simulink model "lab2_EmulationPID_Feedforward"  (R2020b)
settings: Solver=VariableStepAuto  StartTime=0.0  StopTime=10.0  RelTol=1e-3
undefined symbols (not defined in the file): BEMF_Compensator, Beq_hat_final, DiscIntNeverNeededParam, drv, enable_BlackBox, friction_Compensator, gbox, inertia_Compensator, Kd, Ki, Kp, mld, mot, rads2rpm, rpm2rads, sens, tau_sf_hat_final, Tl, Ts
libraries: simulink x1
settings Model: Creator=Musta  LastModifiedBy=Musta

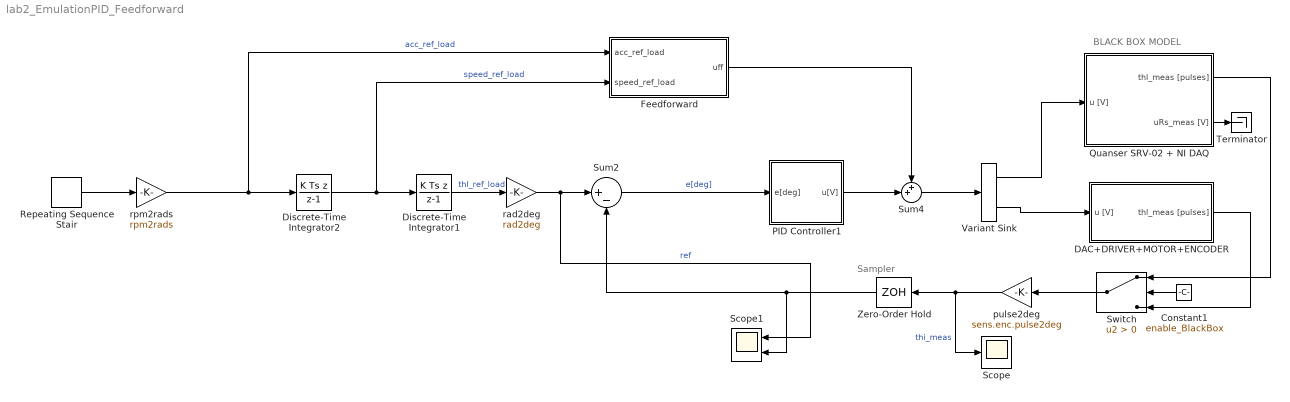
== system lab2_EmulationPID_Feedforward ==
  note: Sampler
  note: BLACK BOX MODEL
  Constant1 : Constant  Value=enable_BlackBox
  DAC+DRIVER+MOTOR+ENCODER : Subsystem
  Discrete-Time Integrator1 : DiscreteIntegrator  IntegratorMethod=Integration: Backward Euler  SampleTime=Ts  ICPrevOutput=DiscIntNeverNeededParam  ICPrevScaledInput=DiscIntNeverNeededParam
  Discrete-Time Integrator2 : DiscreteIntegrator  IntegratorMethod=Integration: Backward Euler  SampleTime=Ts  ICPrevOutput=DiscIntNeverNeededParam  ICPrevScaledInput=DiscIntNeverNeededParam
  Feedforward : Subsystem
  PID Controller1 : Subsystem
  Quanser SRV-02 + NI DAQ : Subsystem  mask(Quanser SRV-02 (with inertial load) + NI DAQ){Ts=Ts, fricType=Karnopp}
      mask prompts: Ts "NI DAQ Sample Time:"; fricType "Friction model"
      mask help: Quanser SRV-02 (with inertial load) + NI DAQ model.
      mask init:
      | %%  Sensors data
      | 
      | %   shunt resistor
      | sens.curr.Rs = 0.5;                         %   resistance [Ohm]   
      | sens.curr.uRs_std = 0.01;                   %   voltage noise standard dev [V]                           
      | sens.curr.uRs_var = sens.curr.uRs_std^2;	%   voltage noise variance [V^2]
      | 
      | %   Hewlett-Packard HEDS-5540#A06 optical encoder
      | sens.enc.ppr = 500*4;                       %   pulses per rotation
      | sens.enc.pulse2deg = 360/sens.enc.ppr;      %   [pulses] -> [deg]
      | sens.enc.pulse2rad = 2*pi/sens.enc.ppr;     %   [pulses] -> [rad]
      | sens.enc.deg2pulse = sens.enc.ppr/360;      %   [deg] -> [pulses]
      | sens.enc.rad2pulse = sens.enc.ppr/2/pi;     %   [rad] -> [pulses]
      | 
      | 
      | %%  Data acquisition board (daq) data
      | 
      | %   NI PCI-6221 DAC data
      | daq.dac.bits = 16;                                  %   resolution (bits)
      | daq.dac.fs   = 10;                                  %   full scale 
      | daq.dac.q    = 2*daq.dac.fs/(2^daq.dac.bits-1);     %	quantization
      | 
      | %   NI PCI-6221 ADC data
      | daq.adc.bits = 16;                                  %   resolution (bits)
      | daq.adc.fs   = 10;                                  %   full scale (as set in SLDRT Analog Input block)
      | daq.adc.q    = 2*daq.adc.fs/(2^daq.adc.bits-1);     %   quantization
      mask Help:
      | Riccardo Antonello (antonello@dei.unipd.it)
      | 
      | April 24, 2020
      | 
      | Dept. of Information Engineering, University of Padova
      mask TypeOptions fricType: Coulomb + viscous | Karnopp
  Repeating Sequence Stair : simulink/Sources/Repeating Sequence Stair  OutValues=[900 0 -900 -900 0 900]  tsamp=0.5  OutMin=[]  OutMax=[]  OutDataTypeStr=double  OutputDataTypeScalingMode=double  OutDataType=fixdt(0,8)  ConRadixGroup=Best Precision: Vector-wise  OutScaling=2^-12
  Scope : Scope
  Scope1 : Scope  NumInputPorts=2
  Sum2 : Sum  Inputs=|+-
  Sum4 : Sum  Inputs=++|
  Switch : Switch  Criteria=u2 > Threshold
  Terminator : Terminator
  Variant Sink : VariantSink
  Zero-Order Hold : ZeroOrderHold  SampleTime=Ts
  pulse2deg : Gain  Gain=sens.enc.pulse2deg
  rad2deg : Gain  Gain=rad2deg
  rpm2rads : Gain  Gain=rpm2rads
  wires:
  PID Controller1/1(u[V]) -> Sum4/2
  Sum2/1 -> PID Controller1/1(e[deg])  "e[deg]"
  Zero-Order Hold/1 -> Scope1/2, Sum2/2
  Feedforward/1(uff) -> Sum4/1
  Discrete-Time Integrator1/1 -> rad2deg/1  "thl_ref_load"
  rpm2rads/1 -> Discrete-Time Integrator2/1, Feedforward/1(acc_ref_load)  "acc_ref_load"
  Discrete-Time Integrator2/1 -> Discrete-Time Integrator1/1, Feedforward/2(speed_ref_load)  "speed_ref_load"
  rad2deg/1 -> Scope1/1, Sum2/1  "ref"
  Repeating Sequence Stair/1 -> rpm2rads/1
  Sum4/1 -> Variant Sink/1
  DAC+DRIVER+MOTOR+ENCODER/1(thl_meas [pulses]) -> Switch/3
  Variant Sink/2 -> DAC+DRIVER+MOTOR+ENCODER/1(u [V])
  Switch/1 -> pulse2deg/1
  Quanser SRV-02 + NI DAQ/1(thl_meas [pulses]) -> Switch/1
  pulse2deg/1 -> Scope/1, Zero-Order Hold/1  "thi_meas"
  Quanser SRV-02 + NI DAQ/2(uRs_meas [V]) -> Terminator/1
  Variant Sink/1 -> Quanser SRV-02 + NI DAQ/1(u [V])
  Constant1/1 -> Switch/2

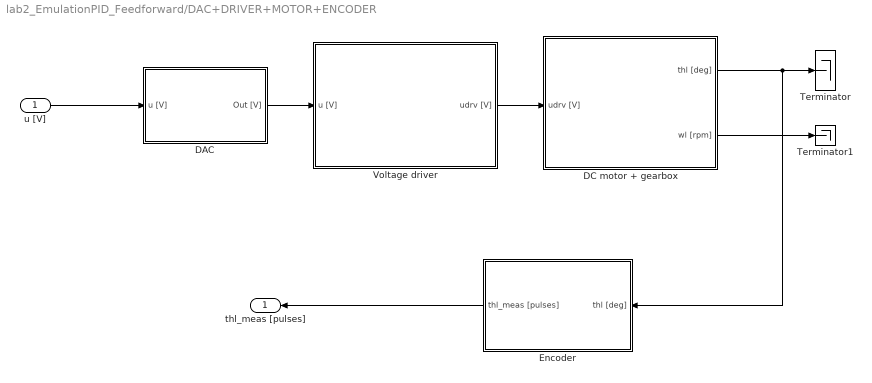
== system lab2_EmulationPID_Feedforward/DAC+DRIVER+MOTOR+ENCODER ==
  u [V] : Inport
  DAC : Subsystem
  DC motor + gearbox : Subsystem
  Encoder : Subsystem
  Terminator : Terminator
  Terminator1 : Terminator
  Voltage driver : Subsystem
  thl_meas [pulses] : Outport
  wires:
  DAC/1(Out [V]) -> Voltage driver/1(u [V])
  DC motor + gearbox/1("thl [deg] ") -> Terminator/1, Encoder/1("thl [deg] ")
  Voltage driver/1(udrv [V]) -> DC motor + gearbox/1(udrv [V])
  DC motor + gearbox/2(wl [rpm]) -> Terminator1/1
  Encoder/1(thl_meas [pulses]) -> thl_meas [pulses]/1
  u [V]/1 -> DAC/1(u [V])

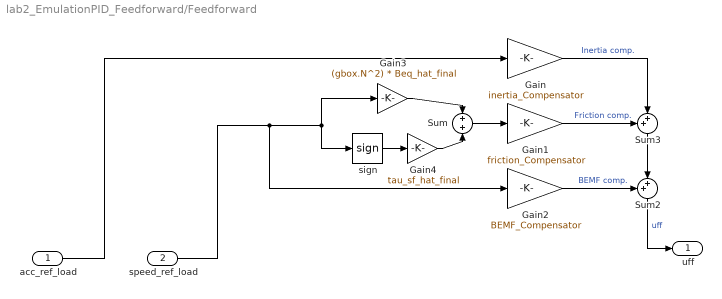
== system lab2_EmulationPID_Feedforward/Feedforward ==
  acc_ref_load : Inport
  speed_ref_load : Inport  Port=2
  Gain : Gain  Gain=inertia_Compensator
  Gain1 : Gain  Gain=friction_Compensator
  Gain2 : Gain  Gain=BEMF_Compensator
  Gain3 : Gain  Gain=(gbox.N^2) * Beq_hat_final
  Gain4 : Gain  Gain=tau_sf_hat_final
  Sum : Sum  Inputs=+|+
  Sum2 : Sum  Inputs=++|
  Sum3 : Sum  Inputs=++|
  sign : Signum
  uff : Outport
  wires:
  sign/1 -> Gain4/1
  Sum/1 -> Gain1/1
  speed_ref_load/1 -> Gain2/1, sign/1, Gain3/1
  Sum3/1 -> Sum2/2
  Gain3/1 -> Sum/1
  Gain/1 -> Sum3/2  "Inertia comp."
  Gain1/1 -> Sum3/1  "Friction comp."
  Gain4/1 -> Sum/2
  Gain2/1 -> Sum2/1  "BEMF comp."
  acc_ref_load/1 -> Gain/1
  Sum2/1 -> uff/1  "uff"

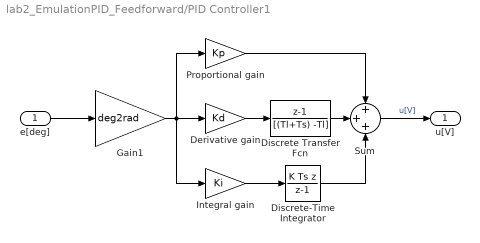
== system lab2_EmulationPID_Feedforward/PID Controller1 ==
  e[deg] : Inport
  Derivative gain : Gain  Gain=Kd
  Discrete Transfer Fcn : DiscreteTransferFcn  Numerator=[1 -1]  Denominator=[(Tl+Ts) -Tl]  SampleTime=Ts
  Discrete-Time Integrator : DiscreteIntegrator  IntegratorMethod=Integration: Backward Euler  SampleTime=Ts  ICPrevOutput=DiscIntNeverNeededParam  ICPrevScaledInput=DiscIntNeverNeededParam
  Gain1 : Gain  Gain=deg2rad
  Integral gain : Gain  Gain=Ki
  Proportional gain : Gain  Gain=Kp
  Sum : Sum  Inputs=+++
  u[V] : Outport
  wires:
  e[deg]/1 -> Gain1/1
  Discrete Transfer Fcn/1 -> Sum/2
  Gain1/1 -> Proportional gain/1, Integral gain/1, Derivative gain/1
  Proportional gain/1 -> Sum/1
  Integral gain/1 -> Discrete-Time Integrator/1
  Discrete-Time Integrator/1 -> Sum/3
  Derivative gain/1 -> Discrete Transfer Fcn/1
  Sum/1 -> u[V]/1  "u[V]"

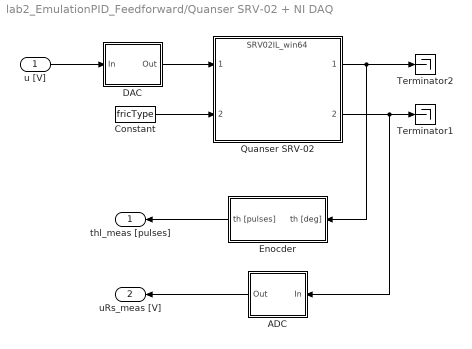
== system lab2_EmulationPID_Feedforward/Quanser SRV-02 + NI DAQ ==
  u [V] : Inport
  ADC : Subsystem
  Constant : Constant  Value=fricType
  DAC : Subsystem
  Enocder : Subsystem
  Quanser SRV-02 : ModelReference  ModelNameDialog=SRV02IL_win64.slxp  ModelReferenceVersion=1.44  CopyOfModelProtected=on
  Terminator1 : Terminator
  Terminator2 : Terminator
  thl_meas [pulses] : Outport
  uRs_meas [V] : Outport  Port=2
  wires:
  Enocder/1(th [pulses]) -> thl_meas [pulses]/1
  ADC/1(Out) -> uRs_meas [V]/1
  DAC/1(Out) -> Quanser SRV-02/1
  Quanser SRV-02/2 -> ADC/1(In), Terminator1/1
  u [V]/1 -> DAC/1(In)
  Quanser SRV-02/1 -> Enocder/1(th [deg]), Terminator2/1
  Constant/1 -> Quanser SRV-02/2

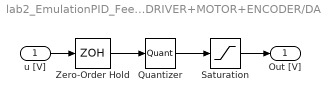
== system lab2_EmulationPID_Feedforward/DAC+DRIVER+MOTOR+ENCODER/DAC ==
  u [V] : Inport
  Quantizer : Quantizer  QuantizationInterval=20/(2^16-1)
  Saturation : Saturate  UpperLimit=10  LowerLimit=-10
  Zero-Order Hold : ZeroOrderHold  SampleTime=Ts
  Out [V] : Outport
  wires:
  u [V]/1 -> Zero-Order Hold/1
  Zero-Order Hold/1 -> Quantizer/1
  Quantizer/1 -> Saturation/1
  Saturation/1 -> Out [V]/1

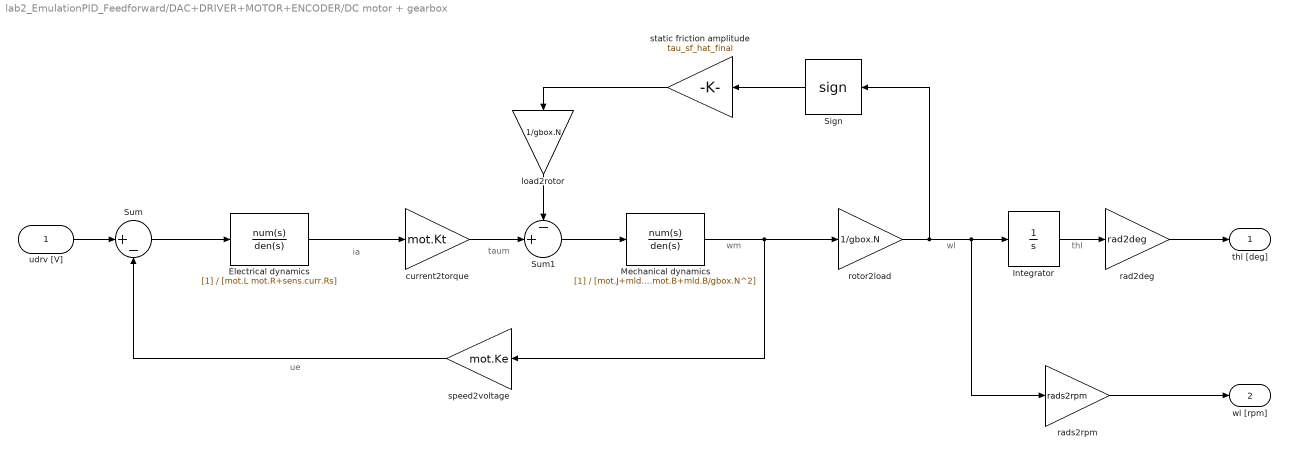
== system lab2_EmulationPID_Feedforward/DAC+DRIVER+MOTOR+ENCODER/DC motor + gearbox ==
  note: thl
  note: wl
  note: wm
  note: ue
  note: taum
  note: ia
  udrv [V] : Inport
  Electrical dynamics : TransferFcn  Denominator=[mot.L mot.R+sens.curr.Rs]
  Integrator : Integrator
  Mechanical dynamics : TransferFcn  Denominator=[mot.J+mld.J/gbox.N^2 mot.B+mld.B/gbox.N^2]
  Sign : Signum  ZeroCross=off
  Sum : Sum  Inputs=|+-
  Sum1 : Sum  Inputs=-+|
  current2torque : Gain  Gain=mot.Kt
  load2rotor : Gain  Gain=1/gbox.N
  rad2deg : Gain  Gain=rad2deg
  rads2rpm : Gain  Gain=rads2rpm
  rotor2load : Gain  Gain=1/gbox.N
  speed2voltage : Gain  Gain=mot.Ke
  static friction amplitude : Gain  Gain=tau_sf_hat_final
  "thl [deg] " : Outport
  wl [rpm] : Outport  Port=2
  wires:
  static friction amplitude/1 -> load2rotor/1
  udrv [V]/1 -> Sum/1
  Electrical dynamics/1 -> current2torque/1
  current2torque/1 -> Sum1/2
  load2rotor/1 -> Sum1/1
  Sign/1 -> static friction amplitude/1
  speed2voltage/1 -> Sum/2
  rad2deg/1 -> "thl [deg] "/1
  Sum1/1 -> Mechanical dynamics/1
  Mechanical dynamics/1 -> speed2voltage/1, rotor2load/1
  rads2rpm/1 -> wl [rpm]/1
  Sum/1 -> Electrical dynamics/1
  rotor2load/1 -> Sign/1, rads2rpm/1, Integrator/1
  Integrator/1 -> rad2deg/1

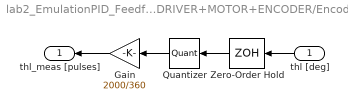
== system lab2_EmulationPID_Feedforward/DAC+DRIVER+MOTOR+ENCODER/Encoder ==
  "thl [deg] " : Inport
  Gain : Gain  Gain=2000/360
  Quantizer : Quantizer  QuantizationInterval=360/(500*4)
  Zero-Order Hold : ZeroOrderHold  SampleTime=Ts
  thl_meas [pulses] : Outport
  wires:
  "thl [deg] "/1 -> Zero-Order Hold/1
  Zero-Order Hold/1 -> Quantizer/1
  Quantizer/1 -> Gain/1
  Gain/1 -> thl_meas [pulses]/1

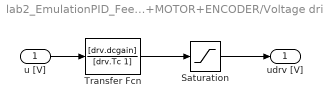
== system lab2_EmulationPID_Feedforward/DAC+DRIVER+MOTOR+ENCODER/Voltage driver ==
  u [V] : Inport
  Saturation : Saturate  UpperLimit=12  LowerLimit=-12
  Transfer Fcn : TransferFcn  Numerator=[drv.dcgain]  Denominator=[drv.Tc 1]
  udrv [V] : Outport
  wires:
  u [V]/1 -> Transfer Fcn/1
  Transfer Fcn/1 -> Saturation/1
  Saturation/1 -> udrv [V]/1

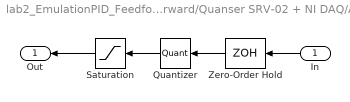
== system lab2_EmulationPID_Feedforward/Quanser SRV-02 + NI DAQ/ADC ==
  In : Inport
  Quantizer : Quantizer  QuantizationInterval=daq.adc.q
  Saturation : Saturate  UpperLimit=daq.adc.fs  LowerLimit=-daq.adc.fs
  Zero-Order Hold : ZeroOrderHold  SampleTime=Ts
  Out : Outport
  wires:
  Saturation/1 -> Out/1
  In/1 -> Zero-Order Hold/1
  Quantizer/1 -> Saturation/1
  Zero-Order Hold/1 -> Quantizer/1

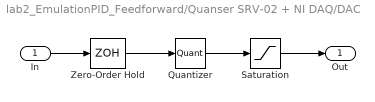
== system lab2_EmulationPID_Feedforward/Quanser SRV-02 + NI DAQ/DAC ==
  In : Inport
  Quantizer : Quantizer  QuantizationInterval=daq.dac.q
  Saturation : Saturate  UpperLimit=daq.dac.fs  LowerLimit=-daq.dac.fs
  Zero-Order Hold : ZeroOrderHold  SampleTime=Ts
  Out : Outport
  wires:
  Quantizer/1 -> Saturation/1
  In/1 -> Zero-Order Hold/1
  Zero-Order Hold/1 -> Quantizer/1
  Saturation/1 -> Out/1

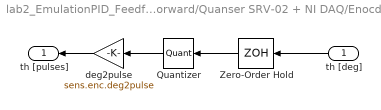
== system lab2_EmulationPID_Feedforward/Quanser SRV-02 + NI DAQ/Enocder ==
  th [deg] : Inport
  Quantizer : Quantizer  QuantizationInterval=sens.enc.pulse2deg
  Zero-Order Hold : ZeroOrderHold  SampleTime=Ts
  deg2pulse : Gain  Gain=sens.enc.deg2pulse
  th [pulses] : Outport
  wires:
  Quantizer/1 -> deg2pulse/1
  th [deg]/1 -> Zero-Order Hold/1
  Zero-Order Hold/1 -> Quantizer/1
  deg2pulse/1 -> th [pulses]/1
